simulink model "E6_5"  (R2023b)
settings: Solver=VariableStepAuto  StartTime=0.0  StopTime=240  RelTol=1e-3
model workspace (MAT data in the model file):
  KLI = Simulink.Parameter
  KLI.Value = 0.01
  KLI.DataType = 'auto'
  KLI.DocUnits = '1/(s^2)'
  KLI.Complexity = 'real'
  KLI.Dimensions = [1 1]
  KLP = Simulink.Parameter
  KLP.Value = 0.5
  KLP.DataType = 'auto'
  KLP.DocUnits = '1/s'
  KLP.Complexity = 'real'
  KLP.Dimensions = [1 1]
  KTI = Simulink.Parameter
  KTI.Value = 0.02
  KTI.DataType = 'auto'
  KTI.DocUnits = '1/s'
  KTI.Complexity = 'real'
  KTI.Dimensions = [1 1]
  KTP = Simulink.Parameter
  KTP.Value = 0.08
  KTP.DataType = 'auto'
  KTP.DocUnits = '1/s'
  KTP.Complexity = 'real'
  KTP.Dimensions = [1 1]
  KWpunto = Simulink.Parameter
  KWpunto.Value = 1.31e-05
  KWpunto.DataType = 'auto'
  KWpunto.DocUnits = 'kg/(s*N)'
  KWpunto.Complexity = 'real'
  KWpunto.Dimensions = [1 1]
  Kni = Simulink.Parameter
  Kni.Value = 0.075
  Kni.DataType = 'auto'
  Kni.DocUnits = '1/s'
  Kni.Complexity = 'real'
  Kni.Dimensions = [1 1]
  L0 = Simulink.Parameter
  L0.Value = 1265519
  L0.DataType = 'auto'
  L0.DocUnits = 'N'
  L0.Complexity = 'real'
  L0.Dimensions = [1 1]
  Tmax = Simulink.Parameter
  Tmax.Value = 320272
  Tmax.DataType = 'auto'
  Tmax.DocUnits = 'N'
  Tmax.Complexity = 'real'
  Tmax.Dimensions = [1 1]
  V0 = Simulink.Parameter
  V0.Value = 178.8
  V0.DataType = 'auto'
  V0.DocUnits = 'm/s'
  V0.Complexity = 'real'
  V0.Dimensions = [1 1]
  Vxe = Simulink.Parameter
  Vxe.Value = 11.176
  Vxe.DataType = 'auto'
  Vxe.DocUnits = 'm/s'
  Vxe.Complexity = 'real'
  Vxe.Dimensions = [1 1]
  Vye = Simulink.Parameter
  Vye.Value = 11.176
  Vye.DataType = 'auto'
  Vye.DocUnits = 'm/s'
  Vye.Complexity = 'real'
  Vye.Dimensions = [1 1]
  Vze = Simulink.Parameter
  Vze.Value = 0
  Vze.DataType = 'auto'
  Vze.DocUnits = 'm/s'
  Vze.Complexity = 'real'
  Vze.Dimensions = [1 1]
  alpha0L = Simulink.Parameter
  alpha0L.Value = -0.050614
  alpha0L.DataType = 'auto'
  alpha0L.DocUnits = 'rad'
  alpha0L.Complexity = 'real'
  alpha0L.Dimensions = [1 1]
  alphaBmax = Simulink.Parameter
  alphaBmax.Value = 8
  alphaBmax.DataType = 'auto'
  alphaBmax.DocUnits = 'deg'
  alphaBmax.Complexity = 'real'
  alphaBmax.Dimensions = [1 1]
  delta0 = Simulink.Parameter
  delta0.Value = 0
  delta0.DataType = 'auto'
  delta0.DocUnits = 'rad'
  delta0.Complexity = 'real'
  delta0.Dimensions = [1 1]
  g = Simulink.Parameter
  g.Value = 9.81
  g.DataType = 'auto'
  g.DocUnits = 'm/(s^2)'
  g.Complexity = 'real'
  g.Dimensions = [1 1]
  gamma0 = Simulink.Parameter
  gamma0.Value = 0
  gamma0.DataType = 'auto'
  gamma0.DocUnits = 'rad'
  gamma0.Complexity = 'real'
  gamma0.Dimensions = [1 1]
  h0 = Simulink.Parameter
  h0.Value = 3048
  h0.DataType = 'auto'
  h0.Complexity = 'real'
  h0.Dimensions = [1 1]
  m0 = Simulink.Parameter
  m0.Value = 129003
  m0.DataType = 'auto'
  m0.DocUnits = 'kg'
  m0.Complexity = 'real'
  m0.Dimensions = [1 1]
  mEmpty = Simulink.Parameter
  mEmpty.Value = 71190
  mEmpty.DataType = 'auto'
  mEmpty.DocUnits = 'kg'
  mEmpty.Complexity = 'real'
  mEmpty.Dimensions = [1 1]
  niMax = Simulink.Parameter
  niMax.Value = 30
  niMax.DataType = 'auto'
  niMax.DocUnits = 'deg'
  niMax.Complexity = 'real'
  niMax.Dimensions = [1 1]
  pL = Simulink.Parameter
  pL.Value = 2.5
  pL.DataType = 'auto'
  pL.DocUnits = 'rad/s'
  pL.Complexity = 'real'
  pL.Dimensions = [1 1]
  pNi = Simulink.Parameter
  pNi.Value = 1
  pNi.DataType = 'auto'
  pNi.DocUnits = 'rad/s'
  pNi.Complexity = 'real'
  pNi.Dimensions = [1 1]
  pT = Simulink.Parameter
  pT.Value = 2
  pT.DataType = 'auto'
  pT.DocUnits = 'rad/s'
  pT.Complexity = 'real'
  pT.Dimensions = [1 1]
  x0 = Simulink.Parameter
  x0.Value = 0
  x0.DataType = 'auto'
  x0.DocUnits = 'm'
  x0.Complexity = 'real'
  x0.Dimensions = [1 1]
  y0 = Simulink.Parameter
  y0.Value = 0
  y0.DataType = 'auto'
  y0.DocUnits = 'm'
  y0.Complexity = 'real'
  y0.Dimensions = [1 1]
values from neighbouring files (symbols this model uses):
  Tmax = Tmax.Values    [displayData.m]
libraries: aerolibconvert2 x5, aerolibatmos2 x1, SignalEditorBlockLib x1
settings Model: Creator=alexl  LastModifiedBy=alexl

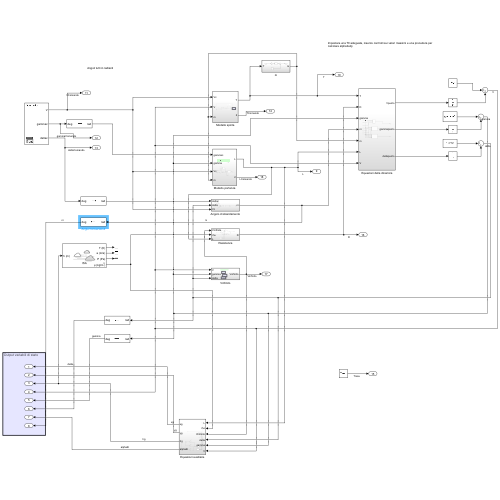
[thumbnail: Simulink's stored preview of the top-level diagram]
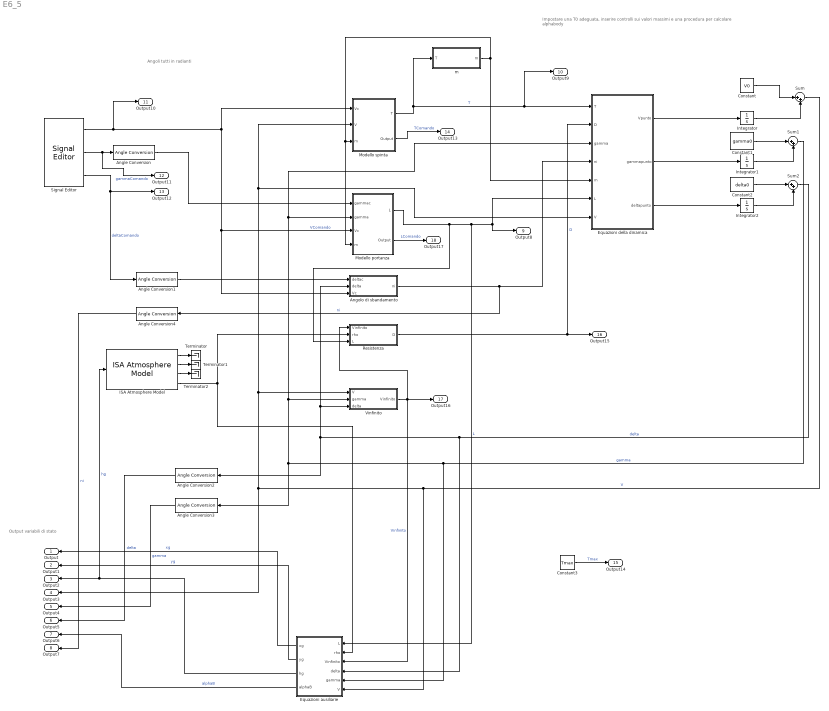
== system E6_5 ==
  note: Output variabili di stato
  note: Impostare una T0 adeguata, inserire controlli sui valori massimi e una procedura per calcolare alphabody
  note: Angoli tutti in radianti
  Angle Conversion : aerolibconvert2/Angle Conversion  IU=deg  OU=rad
  Angle Conversion1 : aerolibconvert2/Angle Conversion  IU=deg  OU=rad
  Angle Conversion2 : aerolibconvert2/Angle Conversion  IU=rad  OU=deg
  Angle Conversion3 : aerolibconvert2/Angle Conversion  IU=rad  OU=deg
  Angle Conversion4 : aerolibconvert2/Angle Conversion  IU=rad  OU=deg
  Angolo di sbandamento : Subsystem
  Constant : Constant  Value=V0
  Constant1 : Constant  Value=gamma0
  Constant2 : Constant  Value=delta0
  Constant3 : Constant  Value=Tmax
  Equazioni ausiliarie : Subsystem
  Equazioni della dinamica : Subsystem
  ISA Atmosphere Model : aerolibatmos2/ISA Atmosphere Model  useExtended=off  action=Warning  custom=off  viscosityOut=off  g=9.80665  gamma=1.4  R=287.0531  L=0.0065  h_trop=11000  h_strat=20000  rho0=1.225  P0=101325  T0=288.15  h0=0
  Integrator : Integrator
  Integrator1 : Integrator
  Integrator2 : Integrator
  Modello portanza : Subsystem
  Modello spinta : Subsystem
  Resistenza : Subsystem
  Signal Editor : SignalEditorBlockLib/Signal Editor  FileName=Scenario.mat  ActiveScenario=Scenario  ActiveSignal=gammac  IsBus=off  OutputBusObjectStr=Bus: BusObject  SampleTime=0  OutputAfterFinalValue=Holding final value  Unit=inherit  PreserveSignalName=on  ApplySigPropsToAllScenarios=on  ApplySigPropsToAllSignals=on
  Sum : Sum  Inputs=|++
  Sum1 : Sum  Inputs=|++
  Sum2 : Sum  Inputs=|++
  Terminator : Terminator
  Terminator1 : Terminator
  Terminator2 : Terminator
  Vinfinito : Subsystem
  m : Subsystem
  Output : Outport
  Output1 : Outport  Port=2
  Output2 : Outport  Port=3
  Output3 : Outport  Port=4
  Output4 : Outport  Port=5
  Output5 : Outport  Port=6
  Output6 : Outport  Port=7
  Output7 : Outport  Port=8
  Output8 : Outport  Port=9
  Output9 : Outport  Port=10
  Output10 : Outport  Port=11
  Output11 : Outport  Port=12
  Output12 : Outport  Port=13
  Output13 : Outport  Port=14
  Output14 : Outport  Port=15
  Output15 : Outport  Port=16
  Output16 : Outport  Port=17
  Output17 : Outport  Port=18
  wires:
  Signal Editor/1 -> Output10/1, Modello spinta/1(Vc), Angolo di sbandamento/3(Vc), Modello portanza/3(Vc)  "VComando"
  Modello spinta/1(T) -> Output9/1, Equazioni della dinamica/1(T), m/1(T)  "T"
  m/1(m) -> Modello portanza/4(m), Modello spinta/3(m), Equazioni della dinamica/5(m)
  Modello portanza/1(L) -> Resistenza/3(L), Equazioni ausiliarie/1(L), Output8/1, Equazioni della dinamica/6(L)  "L"
  Angolo di sbandamento/1(ni) -> Angle Conversion4/1, Equazioni della dinamica/4(ni)  "ni"
  Resistenza/1(D) -> Equazioni della dinamica/2(D), Output15/1  "D"
  Vinfinito/1(Vinfinito) -> Output16/1, Equazioni ausiliarie/3(Vinfinito), Resistenza/1(Vinfinito)  "Vinfinito"
  Equazioni della dinamica/1(Vpunto) -> Integrator/1
  Constant/1 -> Sum/1
  Integrator/1 -> Sum/2
  Sum/1 -> Equazioni ausiliarie/6(V), Output3/1, Equazioni della dinamica/7(V), Modello spinta/2(V), Vinfinito/1(V)  "V"
  Equazioni della dinamica/2(gammapunto) -> Integrator1/1
  Constant1/1 -> Sum1/1
  Integrator1/1 -> Sum1/2
  Integrator2/1 -> Sum2/2
  Constant2/1 -> Sum2/1
  Equazioni della dinamica/3(deltapunto) -> Integrator2/1
  Sum1/1 -> Equazioni ausiliarie/5(gamma), Angle Conversion3/1, Equazioni della dinamica/3(gamma), Modello portanza/2(gamma), Vinfinito/2(gamma)  "gamma"
  Sum2/1 -> Equazioni ausiliarie/4(delta), Angle Conversion2/1, Angolo di sbandamento/2(delta), Vinfinito/3(delta)  "delta"
  ISA Atmosphere Model/4 -> Equazioni ausiliarie/2(rho), Resistenza/2(rho)
  Signal Editor/3 -> Output12/1, Angle Conversion1/1  "deltaComando"
  Angle Conversion/1 -> Modello portanza/1(gammac)
  Angle Conversion1/1 -> Angolo di sbandamento/1(deltac)
  Angle Conversion2/1 -> Output5/1  "delta"
  Angle Conversion3/1 -> Output4/1  "gamma"
  Signal Editor/2 -> Output11/1, Angle Conversion/1  "gammaComando"
  Equazioni ausiliarie/3(hg) -> Output2/1, ISA Atmosphere Model/1  "hg"
  Equazioni ausiliarie/1(xg) -> Output/1  "xg"
  Equazioni ausiliarie/2(yg) -> Output1/1  "yg"
  Equazioni ausiliarie/4(alphaB) -> Output6/1  "alphaB"
  ISA Atmosphere Model/3 -> Terminator2/1
  ISA Atmosphere Model/2 -> Terminator1/1
  ISA Atmosphere Model/1 -> Terminator/1
  Modello spinta/2(Output) -> Output13/1  "TComando"
  Constant3/1 -> Output14/1  "Tmax"
  Modello portanza/2(Output) -> Output17/1  "LComando"
  Angle Conversion4/1 -> Output7/1  "ni"

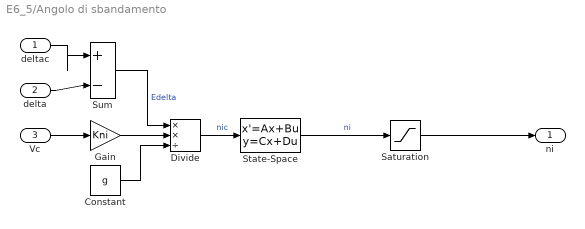
== system E6_5/Angolo di sbandamento ==
  deltac : Inport
  delta : Inport  Port=2
  Vc : Inport  Port=3
  Constant : Constant  Value=g
  Divide : Product  Inputs=**/
  Gain : Gain  Gain=Kni
  Saturation : Saturate  UpperLimit=0.5235  LowerLimit=-0.5235
  State-Space : StateSpace  A=-pNi  B=pNi  D=0  InitialCondition=0
  Sum : Sum  Inputs=|+-
  ni : Outport
  wires:
  deltac/1 -> Sum/1
  State-Space/1 -> Saturation/1  "ni"
  Constant/1 -> Divide/3
  Gain/1 -> Divide/2
  Sum/1 -> Divide/1  "Edelta"
  delta/1 -> Sum/2
  Divide/1 -> State-Space/1  "nic"
  Vc/1 -> Gain/1
  Saturation/1 -> ni/1

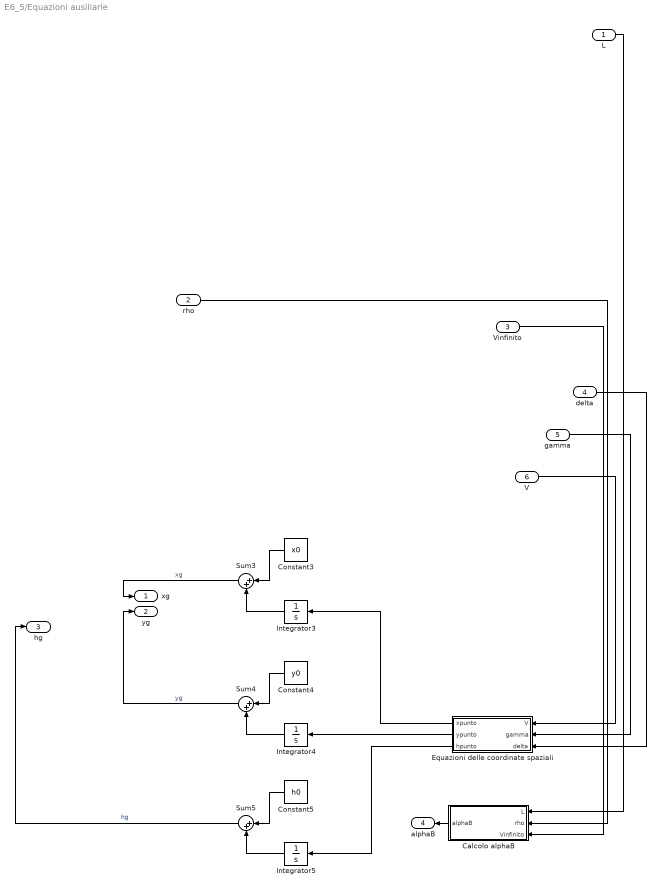
== system E6_5/Equazioni ausiliarie ==
  L : Inport
  rho : Inport  Port=2
  Vinfinito : Inport  Port=3
  delta : Inport  Port=4
  gamma : Inport  Port=5
  V : Inport  Port=6
  Calcolo alphaB : Subsystem
  Constant3 : Constant  Value=x0
  Constant4 : Constant  Value=y0
  Constant5 : Constant  Value=h0
  Equazioni delle coordinate spaziali : Subsystem
  Integrator3 : Integrator
  Integrator4 : Integrator
  Integrator5 : Integrator
  Sum3 : Sum  Inputs=|++
  Sum4 : Sum  Inputs=|++
  Sum5 : Sum  Inputs=|++
  xg : Outport
  yg : Outport  Port=2
  hg : Outport  Port=3
  alphaB : Outport  Port=4
  wires:
  Equazioni delle coordinate spaziali/2(ypunto) -> Integrator4/1
  Equazioni delle coordinate spaziali/1(xpunto) -> Integrator3/1
  Integrator4/1 -> Sum4/2
  Integrator3/1 -> Sum3/2
  Equazioni delle coordinate spaziali/3(hpunto) -> Integrator5/1
  Constant3/1 -> Sum3/1
  Integrator5/1 -> Sum5/2
  Constant4/1 -> Sum4/1
  V/1 -> Equazioni delle coordinate spaziali/1(V)
  Constant5/1 -> Sum5/1
  Sum4/1 -> yg/1  "yg"
  rho/1 -> Calcolo alphaB/2(rho)
  delta/1 -> Equazioni delle coordinate spaziali/3(delta)
  L/1 -> Calcolo alphaB/1(L)
  gamma/1 -> Equazioni delle coordinate spaziali/2(gamma)
  Sum3/1 -> xg/1  "xg"
  Sum5/1 -> hg/1  "hg"
  Calcolo alphaB/1(alphaB) -> alphaB/1
  Vinfinito/1 -> Calcolo alphaB/3(Vinfinito)

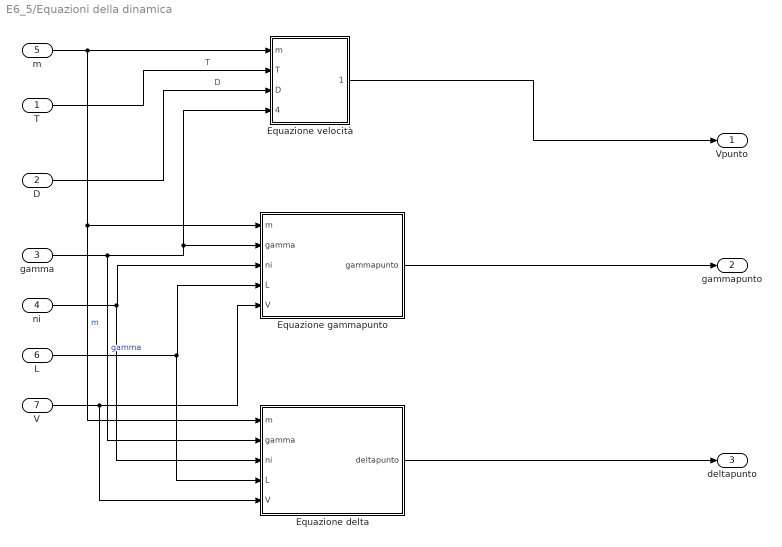
== system E6_5/Equazioni della dinamica ==
  T : Inport
  D : Inport  Port=2
  gamma : Inport  Port=3
  ni : Inport  Port=4
  m : Inport  Port=5
  L : Inport  Port=6
  V : Inport  Port=7
  " Equazione delta" : Subsystem
  Equazione gammapunto : Subsystem
  Equazione velocità : Subsystem
  Vpunto : Outport
  gammapunto : Outport  Port=2
  deltapunto : Outport  Port=3
  wires:
  m/1 -> " Equazione delta"/1(m), Equazione gammapunto/1(m), Equazione velocità/1(m)  "m"
  T/1 -> Equazione velocità/2(T)  "T"
  D/1 -> Equazione velocità/3(D)  "D"
  gamma/1 -> " Equazione delta"/2(gamma), Equazione velocità/4(gamma), Equazione gammapunto/2(gamma)  "gamma"
  ni/1 -> " Equazione delta"/3(ni), Equazione gammapunto/3(ni)
  L/1 -> " Equazione delta"/4(L), Equazione gammapunto/4(L)
  V/1 -> " Equazione delta"/5(V), Equazione gammapunto/5(V)
  Equazione velocità/1(VpuntoSubs) -> Vpunto/1
  Equazione gammapunto/1(gammapunto) -> gammapunto/1
  " Equazione delta"/1(deltapunto) -> deltapunto/1

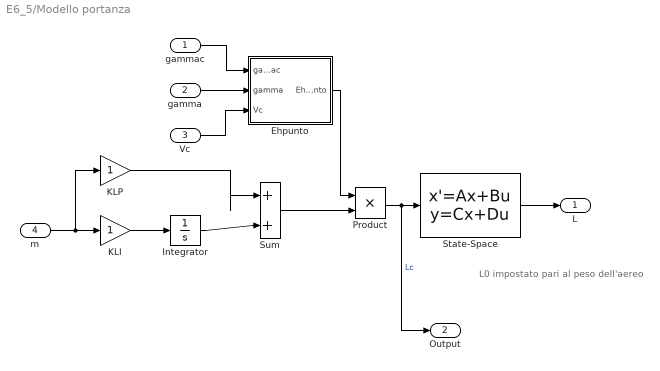
== system E6_5/Modello portanza ==
  note: L0 impostato pari al peso dell'aereo
  gammac : Inport
  gamma : Inport  Port=2
  Vc : Inport  Port=3
  m : Inport  Port=4
  Ehpunto : Subsystem
  Integrator : Integrator
  KLI : Gain
  KLP : Gain
  Product : Product
  State-Space : StateSpace  A=-pL  B=pL  D=0  InitialCondition=L0
  Sum : Sum  Inputs=|++
  L : Outport
  Output : Outport  Port=2
  wires:
  Integrator/1 -> Sum/2
  KLI/1 -> Integrator/1
  KLP/1 -> Sum/1
  m/1 -> KLI/1, KLP/1
  gamma/1 -> Ehpunto/2(gamma)
  gammac/1 -> Ehpunto/1(gammac)
  Vc/1 -> Ehpunto/3(Vc)
  Ehpunto/1(Ehpunto) -> Product/1
  Sum/1 -> Product/2
  Product/1 -> Output/1, State-Space/1  "Lc"
  State-Space/1 -> L/1

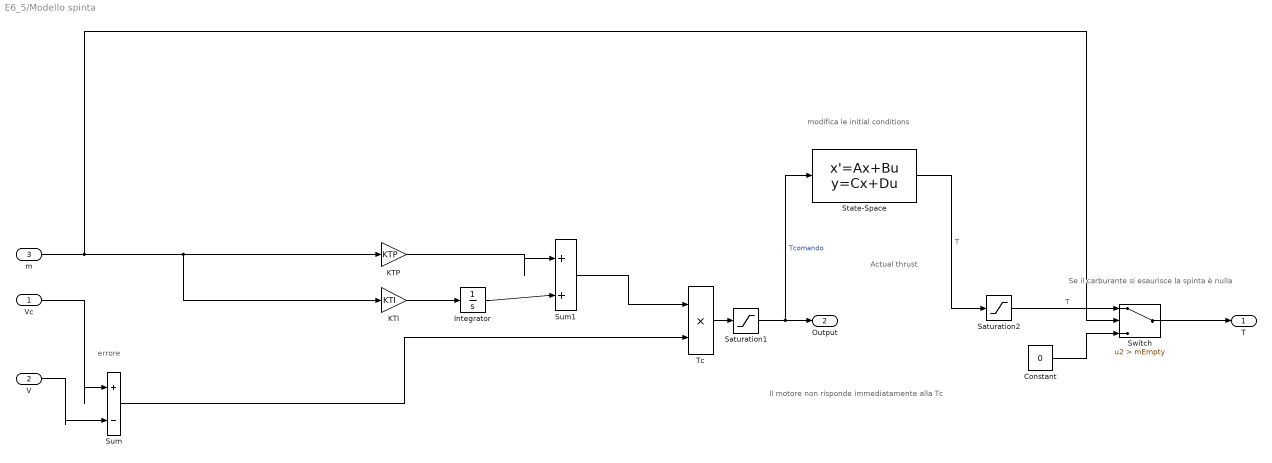
== system E6_5/Modello spinta ==
  note: Se il carburante si esaurisce la spinta è nulla
  note: Actual thrust
  note: modifica le initial conditions
  note: Il motore non risponde immediatamente alla Tc
  note: errore
  Vc : Inport
  V : Inport  Port=2
  m : Inport  Port=3
  Constant : Constant  Value=0
  Integrator : Integrator
  KTI : Gain  Gain=KTI
  KTP : Gain  Gain=KTP
  Saturation1 : Saturate  UpperLimit=Tmax  LowerLimit=0
  Saturation2 : Saturate  UpperLimit=Tmax  LowerLimit=0
  State-Space : StateSpace  A=-pT  B=pT  D=0  InitialCondition=0
  Sum : Sum  Inputs=|+-
  Sum1 : Sum  Inputs=|++
  Switch : Switch  Criteria=u2 > Threshold  Threshold=mEmpty  SaturateOnIntegerOverflow=off  InputSameDT=off
  Tc : Product
  T : Outport
  Output : Outport  Port=2
  wires:
  Vc/1 -> Sum/1
  V/1 -> Sum/2
  m/1 -> Switch/2, KTI/1, KTP/1
  KTI/1 -> Integrator/1
  Integrator/1 -> Sum1/2
  KTP/1 -> Sum1/1
  Sum1/1 -> Tc/1
  Sum/1 -> Tc/2
  State-Space/1 -> Saturation2/1  "T"
  Constant/1 -> Switch/3
  Switch/1 -> T/1
  Tc/1 -> Saturation1/1
  Saturation1/1 -> Output/1, State-Space/1  "Tcomando"
  Saturation2/1 -> Switch/1  "T"

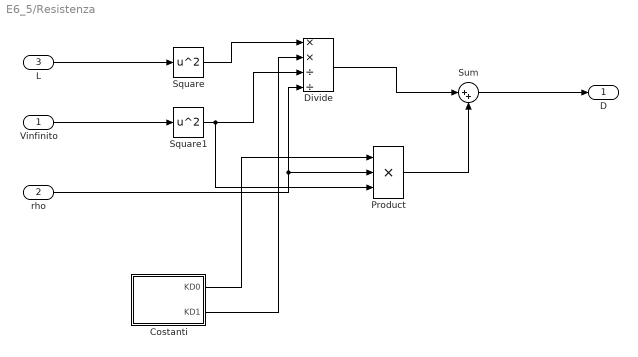
== system E6_5/Resistenza ==
  Vinfinito : Inport
  rho : Inport  Port=2
  L : Inport  Port=3
  Costanti : MATLAB Function  TreatAsAtomicUnit=on
  Divide : Product  Inputs=**//
  Product : Product  Inputs=3
  Square : Math  Operator=square
  Square1 : Math  Operator=square
  Sum : Sum  Inputs=|++
  D : Outport
  wires:
  L/1 -> Square/1
  Square/1 -> Divide/1
  Square1/1 -> Product/3, Divide/3
  Costanti/2(KD1) -> Divide/2
  rho/1 -> Product/2, Divide/4
  Costanti/1(KD0) -> Product/1
  Divide/1 -> Sum/1
  Product/1 -> Sum/2
  Sum/1 -> D/1
  Vinfinito/1 -> Square1/1

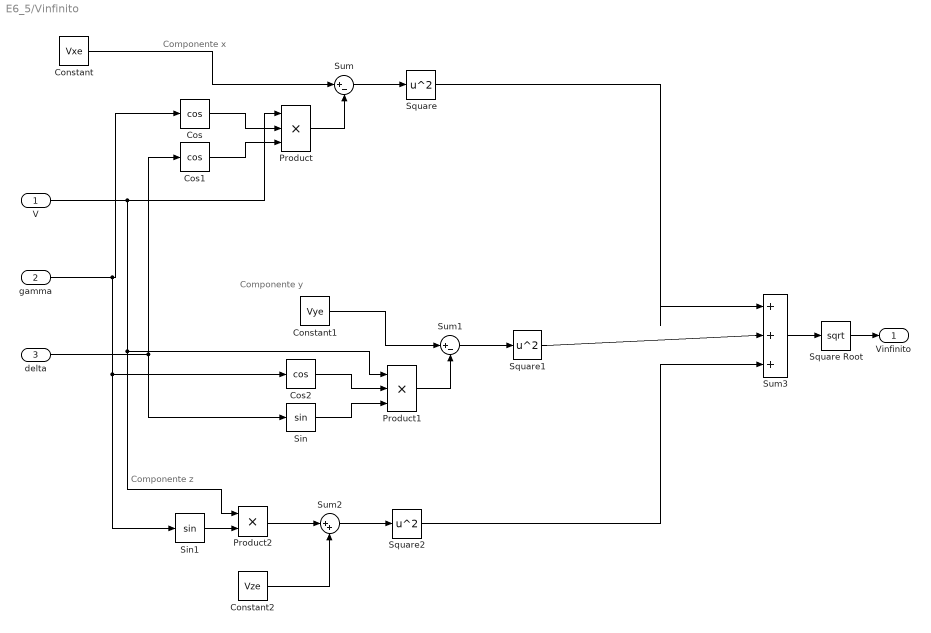
== system E6_5/Vinfinito ==
  note: Componente z
  note: Componente y
  note: Componente x
  V : Inport
  gamma : Inport  Port=2
  delta : Inport  Port=3
  Constant : Constant  Value=Vxe
  Constant1 : Constant  Value=Vye
  Constant2 : Constant  Value=Vze
  Cos : Trigonometry  Operator=cos
  Cos1 : Trigonometry  Operator=cos
  Cos2 : Trigonometry  Operator=cos
  Product : Product  Inputs=3
  Product1 : Product  Inputs=3
  Product2 : Product
  Sin : Trigonometry
  Sin1 : Trigonometry
  Square : Math  Operator=square
  Square Root : Sqrt
  Square1 : Math  Operator=square
  Square2 : Math  Operator=square
  Sum : Sum  Inputs=|+-
  Sum1 : Sum  Inputs=|+-
  Sum2 : Sum  Inputs=|++
  Sum3 : Sum  Inputs=|+++
  Vinfinito : Outport
  wires:
  gamma/1 -> Sin1/1, Cos2/1, Cos/1
  delta/1 -> Cos1/1, Sin/1
  Cos1/1 -> Product/3
  Cos/1 -> Product/2
  V/1 -> Product2/1, Product1/1, Product/1
  Constant/1 -> Sum/1
  Product/1 -> Sum/2
  Sum/1 -> Square/1
  Sin/1 -> Product1/3
  Constant1/1 -> Sum1/1
  Product1/1 -> Sum1/2
  Cos2/1 -> Product1/2
  Sum1/1 -> Square1/1
  Sin1/1 -> Product2/2
  Product2/1 -> Sum2/1
  Sum2/1 -> Square2/1
  Constant2/1 -> Sum2/2
  Square/1 -> Sum3/1
  Square1/1 -> Sum3/2
  Square2/1 -> Sum3/3
  Sum3/1 -> Square Root/1
  Square Root/1 -> Vinfinito/1

== system E6_5/m ==
  T : Inport
  Constant : Constant  Value=m0
  Gain : Gain  Gain=-KWpunto
  Integrator : Integrator
  Sum : Sum  Inputs=|++
  m : Outport
  wires:
  Sum/1 -> m/1
  T/1 -> Gain/1
  Gain/1 -> Integrator/1
  Integrator/1 -> Sum/1
  Constant/1 -> Sum/2

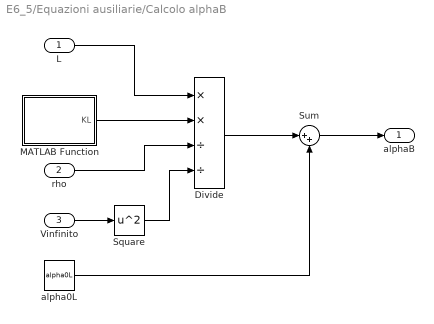
== system E6_5/Equazioni ausiliarie/Calcolo alphaB ==
  L : Inport
  rho : Inport  Port=2
  Vinfinito : Inport  Port=3
  Divide : Product  Inputs=**//
  MATLAB Function : MATLAB Function  TreatAsAtomicUnit=on
  Square : Math  Operator=square
  Sum : Sum  Inputs=|++
  alpha0L : Constant  Value=alpha0L
  alphaB : Outport
  wires:
  L/1 -> Divide/1
  MATLAB Function/1(KL) -> Divide/2
  rho/1 -> Divide/3
  Vinfinito/1 -> Square/1
  Square/1 -> Divide/4
  Divide/1 -> Sum/1
  alpha0L/1 -> Sum/2
  Sum/1 -> alphaB/1

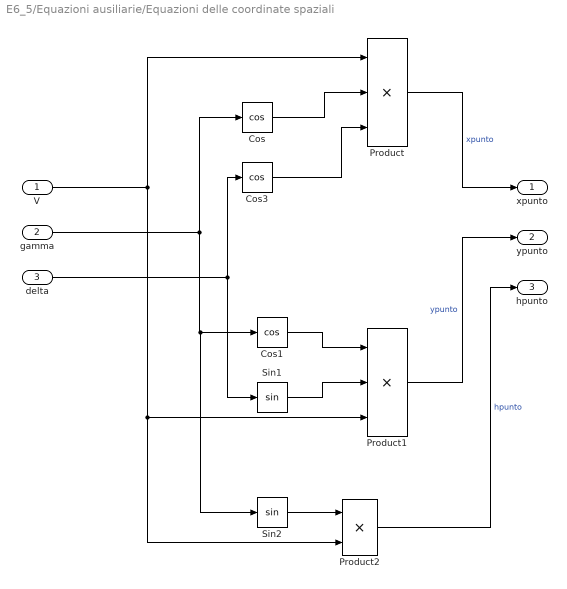
== system E6_5/Equazioni ausiliarie/Equazioni delle coordinate spaziali ==
  V : Inport
  gamma : Inport  Port=2
  delta : Inport  Port=3
  Cos : Trigonometry  Operator=cos
  Cos1 : Trigonometry  Operator=cos
  Cos3 : Trigonometry  Operator=cos
  Product : Product  Inputs=3
  Product1 : Product  Inputs=3
  Product2 : Product
  Sin1 : Trigonometry
  Sin2 : Trigonometry
  xpunto : Outport
  ypunto : Outport  Port=2
  hpunto : Outport  Port=3
  wires:
  Cos3/1 -> Product/3
  Cos/1 -> Product/2
  V/1 -> Product2/2, Product1/3, Product/1
  gamma/1 -> Sin2/1, Cos1/1, Cos/1
  delta/1 -> Sin1/1, Cos3/1
  Product/1 -> xpunto/1  "xpunto"
  Cos1/1 -> Product1/1
  Sin1/1 -> Product1/2
  Product1/1 -> ypunto/1  "ypunto"
  Sin2/1 -> Product2/1
  Product2/1 -> hpunto/1  "hpunto"

== system E6_5/Equazioni della dinamica/ Equazione delta ==
  m : Inport
  gamma : Inport  Port=2
  ni : Inport  Port=3
  L : Inport  Port=4
  V : Inport  Port=5
  Cos : Trigonometry  Operator=cos
  Divide : Product  Inputs=**///
  Sin : Trigonometry
  deltapunto : Outport
  wires:
  V/1 -> Divide/4
  L/1 -> Divide/1
  Cos/1 -> Divide/3
  Sin/1 -> Divide/2
  gamma/1 -> Cos/1
  ni/1 -> Sin/1
  Divide/1 -> deltapunto/1  "deltapunto"
  m/1 -> Divide/5

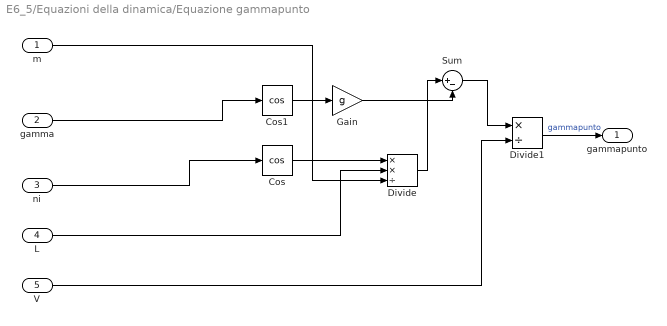
== system E6_5/Equazioni della dinamica/Equazione gammapunto ==
  m : Inport
  gamma : Inport  Port=2
  ni : Inport  Port=3
  L : Inport  Port=4
  V : Inport  Port=5
  Cos : Trigonometry  Operator=cos
  Cos1 : Trigonometry  Operator=cos
  Divide : Product  Inputs=**/
  Divide1 : Product  Inputs=*/
  Gain : Gain  Gain=g
  Sum : Sum  Inputs=|+-
  gammapunto : Outport
  wires:
  gamma/1 -> Cos1/1
  ni/1 -> Cos/1
  Cos/1 -> Divide/1
  Sum/1 -> Divide1/1
  Cos1/1 -> Gain/1
  L/1 -> Divide/2
  m/1 -> Divide/3
  V/1 -> Divide1/2
  Divide1/1 -> gammapunto/1  "gammapunto"
  Gain/1 -> Sum/2
  Divide/1 -> Sum/1

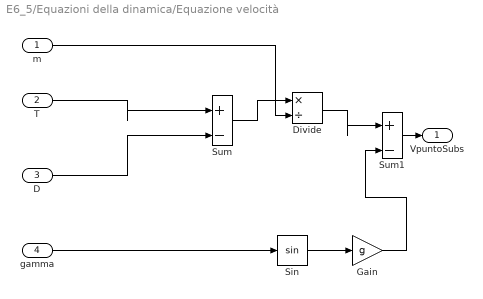
== system E6_5/Equazioni della dinamica/Equazione velocità ==
  m : Inport
  T : Inport  Port=2
  D : Inport  Port=3
  gamma : Inport  Port=4
  Divide : Product  Inputs=*/
  Gain : Gain  Gain=g
  Sin : Trigonometry
  Sum : Sum  Inputs=|+-
  Sum1 : Sum  Inputs=|+-
  VpuntoSubs : Outport
  wires:
  T/1 -> Sum/1
  m/1 -> Divide/2
  Divide/1 -> Sum1/1
  Gain/1 -> Sum1/2
  Sum/1 -> Divide/1
  Sin/1 -> Gain/1
  gamma/1 -> Sin/1
  D/1 -> Sum/2
  Sum1/1 -> VpuntoSubs/1

== system E6_5/Modello portanza/Ehpunto ==
  gammac : Inport
  gamma : Inport  Port=2
  Vc : Inport  Port=3
  Product : Product
  Sin : Trigonometry
  Sin1 : Trigonometry
  Sum : Sum  Inputs=|+-
  Ehpunto : Outport
  wires:
  Sin1/1 -> Sum/1
  Sin/1 -> Sum/2
  gammac/1 -> Sin1/1
  gamma/1 -> Sin/1
  Sum/1 -> Product/1
  Vc/1 -> Product/2
  Product/1 -> Ehpunto/1

== matlab function E6_5/Resistenza/Costanti ==
  data: KD0 output; KD1 output
function [KD0, KD1] = fcn()
    S=280;
    AR=7.082;
    CD0=0.020;
    eff=0.95;
    KD0=0.5*S*CD0;
    KD1=2/(S*pi*AR*eff);
end

== matlab function E6_5/Equazioni ausiliarie/Calcolo alphaB/MATLAB Function ==
  data: KL output
function KL = fcn()
S=280;
CLalpha=5.73;
KL=2/(S*CLalpha);
